simulink model "Q1_W3"  (R2020b)
settings: Solver=VariableStepAuto  StartTime=0.0  StopTime=10.0  RelTol=1e-3
settings Model: Creator=hp  LastModifiedBy=hp

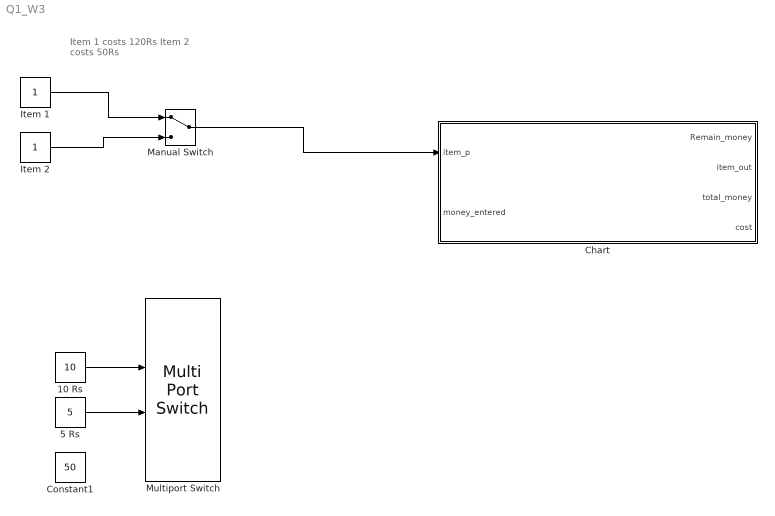
== system Q1_W3 ==
  note: Item 1 costs 120Rs
      | Item 2 costs  50Rs
  10 Rs : Constant  Value=10
  5 Rs : Constant  Value=5
  Chart : Stateflow chart  TreatAsAtomicUnit=on
  Constant1 : Constant  Value=50
  Item 1 : Constant
  Item 2 : Constant
  Manual Switch : ManualSwitch
  Multiport Switch : MultiPortSwitch
  wires:
  10 Rs/1 -> Multiport Switch/2
  5 Rs/1 -> Multiport Switch/3
  Manual Switch/1 -> Chart/1(item_p)
  Item 1/1 -> Manual Switch/1
  Item 2/1 -> Manual Switch/2

== stateflow chart Q1_W3/Chart ==
  state zeroState
    total_money=0;
  state Item
  state moneyState
    entry:
    total_money=total_money+money_entered;
    money_entered=0;
  state itemOutput
    Remain_money=total_money-cost;
  (default) -> zeroState
  zeroState -> Item [order 1] : [item_p==1]{cost=120;}
  zeroState -> Item [order 2] : [item_p==2]{cost=50}
  itemOutput -> zeroState : [item_out==1]{total_money=0;item_out=0;}
  Item -> moneyState : [(money_entered>0)&&(item_out==0)]
  moneyState -> Item [order 1] : [(total_money<cost)&&(item_out==0)]
  moneyState -> itemOutput [order 2] : [total_money>cost]{item_out=1;}
  data: item_p input; Remain_money output; item_out output; total_money output; money_entered input; cost output
